simulink model "ControlDes"  (R2026a)
settings: Solver=ode3  StopTime=4  FixedStep=0.001  EnableMultiTasking=on
(part 8 of 12)

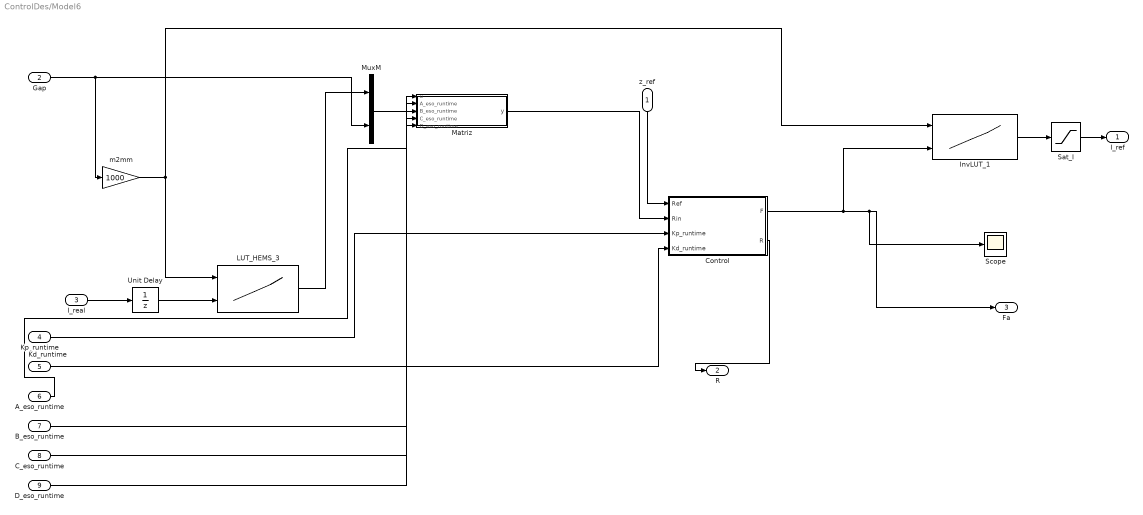
== system ControlDes/Model6 ==
  z_ref : Inport
  Gap : Inport  Port=2
  I_real : Inport  Port=3
  Kp_runtime : Inport  Port=4  OutDataTypeStr=double
  Kd_runtime : Inport  Port=5  OutDataTypeStr=double
  A_eso_runtime : Inport  Port=6  OutDataTypeStr=double  PortDimensions=[3 3]
  B_eso_runtime : Inport  Port=7  OutDataTypeStr=double  PortDimensions=[3 2]
  C_eso_runtime : Inport  Port=8  OutDataTypeStr=double  PortDimensions=[3 3]
  D_eso_runtime : Inport  Port=9  OutDataTypeStr=double  PortDimensions=[3 2]
  Control : Subsystem
  InvLUT_1 : Lookup_n-D  BreakpointsForDimension1=[0.5 1 1.5 2 2.5 3 3.5 4 4.5 5 5.5 6 6.5 7 7.5 8 8.5 9 9.5 10 10.5 11 11.5 12 12.5 13 13.5 14 14.5 15 15.5 16 16.5]  BreakpointsForDimension2=[0 38.719701974874376 77.439403949748751 116.15910592462312 154.8788078994975 193.59850987437187 232.31821184924624 271.03791382412061 309.757615798995 348.47731777386934 387.19701974874374 425.91672172361808 464.63642369849248 503.35612567336682 542.07582764824122 580.79552962311561 619.51523159799001 658.23493357286429 696.95463554773869 735.67433752261297 774.39403949748748 813.11374147236188 851.83344344723616 890.55314542211056 929.27284739698496 967.99254937185924 1006.7122513467336 1045.431953321608 1084.1516552964824 1122.8713572713568 1161.5910592462312 1200.3107612211056 1239.03046319598 1277.7501651708544 1316.4698671457286 1355.189569120603 1393.9092710954774 1432.628973070352 1471.3486750452259 1510.0683770201006 1548.788078994975 1587.5077809698494 1626.2274829447238 1664.9471849195982 1703.6668868944723 1742.3865888693467 1781.1062908442211 1819.8259928190955 1858.5456947939699 1897.2653967688443 1935.9850987437185 1974.7048007185929 2013.4245026934673 2052.1442046683419 2090.8639066432161 2129.5836086180907 2168.3033105929649 2207.023012567839 2245.7427145427137 2284.4624165175878 2323.1821184924625 2361.9018204673371 2400.6215224422112 2439.3412244170854 2478.06092639196 2516.7806283668342 2555.5003303417088 2594.220032316583 2632.9397342914572 2671.6594362663318 2710.379138241206 2749.0988402160806 2787.8185421909548 2826.5382441658294 2865.257946140704 2903.9776481155782 2942.6973500904519 2981.4170520653265 3020.1367540402011 3058.8564560150753 3097.5761579899499 3136.2958599648241 3175.0155619396987 3213.7352639145729 3252.4549658894475 3291.1746678643217 3329.8943698391963 3368.6140718140709 3407.3337737889447 3446.0534757638188 3484.7731777386934 3523.4928797135676 3562.2125816884422 3600.9322836633169 3639.651985638191 3678.3716876130657 3717.0913895879398 3755.8110915628145 3794.5307935376886 3833.2504955125628 3871.970197487437 3910.6898994623116 3949.4096014371858 3988.1293034120604 4026.8490053869346 4065.5687073618092 4104.2884093366838 4143.0081113115584 4181.7278132864321 4220.4475152613068 4259.1672172361814 4297.8869192110551 4336.6066211859297 4375.3263231608043 4414.0460251356781 4452.7657271105527 4491.4854290854273 4530.2051310603019 4568.9248330351757 4607.6445350100503 4646.3642369849249 4685.0839389597995 4723.8036409346741 4762.5233429095479 4801.2430448844225 4839.9627468592962 4878.6824488341708 4917.4021508090455 4956.1218527839201 4994.8415547587938 5033.5612567336684 5072.280958708543 5111.0006606834177 5149.7203626582923 5188.440064633166 5227.1597666080397 5265.8794685829143 5304.5991705577899 5343.3188725326636 5382.0385745075382 5420.7582764824119 5459.4779784572856 5498.1976804321612 5536.9173824070349 5575.6370843819095 5614.3567863567841 5653.0764883316588 5691.7961903065325 5730.515892281408 5769.2355942562817 5807.9552962311564 5846.6749982060301 5885.3947001809038 5924.1144021557793 5962.834104130653 6001.5538061055277 6040.2735080804023 6078.9932100552769 6117.7129120301506 6156.4326140050252 6195.1523159798999 6233.8720179547745 6272.5917199296482 6311.3114219045219 6350.0311238793975 6388.7508258542712 6427.4705278291458 6466.1902298040195 6504.909931778895 6543.6296337537688 6582.3493357286434 6621.069037703518 6659.7887396783926 6698.5084416532663 6737.2281436281419 6775.9478456030156 6814.6675475778893 6853.3872495527639 6892.1069515276376 6930.8266535025132 6969.5463554773869 7008.2660574522615 7046.9857594271352 7085.7054614020108 7124.4251633768845 7163.1448653517591 7201.8645673266337 7240.5842693015074 7279.3039712763821 7318.0236732512558 7356.7433752261313 7395.463077201005 7434.1827791758797 7472.9024811507534 7511.6221831256289 7550.3418851005026 7589.0615870753772 7627.7812890502519 7666.5009910251256 7705.2206930000002]  Table=[0 0.20825445101853096 0.41650890203706192 0.62476335305559283 0.83301780407412385 1.0135826468062146 1.082118922511446 1.1506551982166775 1.219191473921909 1.2877277496271402 1.3562640253323717 1.4248003010376031 1.4933365767428346 1.5618728524480658 1.6304091281532973 1.6989454038585288 1.7674816795637602 1.8360179552689915 1.9045542309742229 1.9730905066794542 2.0259914205399863 2.0687849073782689 2.1115783942165511 2.1543718810548338 2.1971653678931164 2.2399588547313991 2.2827523415696813 2.325545828407964 2.3683393152462466 2.4111328020845288 2.4539262889228119 2.4967197757610946 2.5395132625993773 2.5823067494376595 2.6251002362759417 2.6678937231142243 2.710687209952507 2.7534806967907901 2.7962741836290719 2.839067670467355 2.8818611573056376 2.9246546441439203 2.9674481309822025 3.0082039458877476 3.0424832420422163 3.076762538196685 3.1110418343511541 3.1453211305056232 3.1796004266600919 3.2138797228145606 3.2481590189690297 3.2824383151234988 3.3167176112779675 3.3509969074324366 3.3852762035869057 3.4195554997413744 3.4538347958958431 3.4881140920503118 3.5223933882047813 3.55667268435925 3.5909519805137191 3.6252312766681882 3.6595105728226569 3.6937898689771256 3.7280691651315947 3.7623484612860634 3.7966277574405325 3.8309070535950012 3.8651863497494698 3.8994656459039394 3.9337449420584081 3.9680242382128772 4.0026883536532365 4.0426942126296082 4.0827000716059798 4.1227059305823506 4.1627117895587222 4.2027176485350939 4.2427235075114647 4.2827293664878363 4.3227352254642071 4.3627410844405787 4.4027469434169504 4.4427528023933212 4.4827586613696928 4.5227645203460636 4.5627703793224352 4.6027762382988069 4.6427820972751777 4.6827879562515484 4.7227938152279201 4.7627996742042917 4.8028055331806625 4.842811392157035 4.8828172511334049 4.9228231101097766 4.9628289690861482 5.004895171693434 5.0739771562489926 5.1430591408045503 5.212141125360108 5.2812231099156675 5.350305094471226 5.4193870790267855 5.4884690635823423 5.5575510481379027 5.6266330326934613 5.6957150172490207 5.7647970018045775 5.8338789863601361 5.9029609709156956 5.9720429554712533 6.060635964208382 6.1624927143999662 6.2643494645915485 6.3662062147831326 6.4680629649747168 6.5699197151663018 6.6717764653578833 6.7736332155494674 6.8754899657410515 6.9773467159326366 7.1052458067439899 7.2405933662740365 7.3759409258040867 7.5112884853341342 7.6466360448641844 7.7819836043942345 7.9173311639242847 8.0581390909222392 8.2075159845450063 8.3568928781677734 8.5062697717905404 8.6556466654133075 8.8050235590360693 8.9544004526588328 9.1109942620640414 9.2707591690610673 9.430524076058088 9.5902889830551104 9.7500538900521292 9.909818797049148 10.07860600232517 10.259086199851795 10.439566397378425 10.620046594905055 10.800526792431686 10.981006989958312 11.179637509673544 11.380402745194747 11.581167980715957 11.781933216237162 11.982698451758367 12.200814130096445 12.420566042437333 12.640317954778226 12.860069867119119 13.126007972843706 13.472911953059718 13.819815933275743 14.248324772175067 14.765028806201716 15.318870467347217 15.903685701086824 16.530613286533896 17.178435440269205 17.861895428989815 18.58639634639496 19.342319000305999 20.130582236557807 20.946504242050416 21.793465366913725 22.66596895426494 23.559530190599418 24.471656612462336 25.40419986962144 26.362632409957975 27.351818955653389 28.373533575187398 29.440672985292188 30.570327923183555 31.757263294366073 32.986746804015425 34.246450693164164 35.52223706959721 36.807114490416751 38.099172703380667 39.396598812923777 40.695909456634084 41.995762806636158 43.296542367305818 44.597395639785859 45.898496497631839 47.199521876773268 48.499918470691156 49.80095993571296 51.101605949724835 52.401915628484389 53.701245517447497 55;0 0.76888357898292115 1.1751199837457729 1.4255013576533873 1.6758827315610019 1.9262641054686163 2.1058823348051132 2.2559623966027069 2.4060424584003006 2.5561225201978948 2.706202581995488 2.8562826437930822 3.0045785783675409 3.1125756111632508 ...(+52833 chars)]  ExtrapMethod=Clip  InternalRulePriority=Speed  RndMeth=Simplest
      settings: InputPortMap=u0,u1
  LUT_HEMS_3 : Lookup_n-D  BreakpointsForDimension1=[0.5 1 1.5 2 2.5 3 3.5 4 4.5 5 5.5 6 6.5 7 7.5 8 8.5 9 9.5 10 10.5 11 11.5 12 12.5 13 13.5 14 14.5 15 15.5 16 16.5]  BreakpointsForDimension2=[0 1 2 3 4 5 6 7 8 9 10 11 12 13 14 15 16 17 18 19 20 21 22 23 24 25 26 27 28 29 30 31 32 33 34 35 36 37 38 39 40 41 42 43 44 45 46 47 48 49 50 51 52 53 54 55]  Table=[0 185.9249672 750.87690799999996 1655.6805320000001 2785.216617 3753.0674009999998 4313.5565390000002 4693.6953309999999 4979.7714310000001 5238.9795389999999 5481.3337750000001 5695.8708960000004 5888.731487 6064.928825 6176.543866 6251.4798049999999 6317.6882409999998 6378.6420159999998 6435.2944939999998 6487.981957 6537.4328340000002 6584.8879850000003 6630.4867649999997 6674.4857750000001 6717.4194129999996 6759.4176170000001 6800.3137919999999 6839.8959009999999 6878.2433190000002 6915.358142 6950.460161 6983.9254600000004 7016.0683060000001 7047.4010179999996 7078.2087309999997 7108.6275150000001 7138.8774709999998 7168.9443259999998 7198.9040859999996 7228.755862 7258.5804779999999 7288.3594860000003 7318.1499009999998 7347.9142069999998 7377.6879230000004 7407.4423319999996 7437.2036580000004 7466.9636659999996 7496.7288989999997 7526.5203250000004 7556.2615880000003 7586.0370910000001 7615.8040099999998 7645.6044910000001 7675.4036120000001 7705.2206930000002;0 50.358341670000001 205.00124249999999 462.99488609999997 821.52049529999999 1275.4488719999999 1815.4468879999999 2417.3712139999998 3013.984723 3491.2876780000001 3838.5691499999998 4118.0858349999999 4346.8618219999998 4558.9346269999996 4759.0309299999999 4942.0177089999997 5105.9639639999996 5253.0348219999996 5362.5162200000004 5440.8379949999999 5509.7998870000001 5572.7200860000003 5632.2593720000004 5689.6635800000004 5744.5173999999997 5797.501671 5848.7229440000001 5898.1835080000001 5945.531156 5990.6949679999998 6033.8417140000001 6075.4827839999998 6116.2033110000002 6156.1693610000002 6195.5075500000003 6234.0945689999999 6271.969083 6309.1572560000004 6345.8601040000003 6382.0602360000003 6417.9799970000004 6453.7335750000002 6489.4389899999996 6524.967318 6560.4583140000004 6595.8979929999996 6631.2596970000004 6666.589696 6701.9197940000004 6737.2543530000003 6772.5132160000003 6807.4936710000002 6842.7713949999998 6878.0320149999998 6913.2557580000002 6948.244514;0 23.217442720000001 94.340941790000002 213.54810789999999 380.32169820000001 594.10779100000002 853.75137949999998 1157.775693 1503.429785 1885.7072029999999 2292.655694 2695.2178359999998 3047.2340450000002 3333.626076 3570.0121479999998 3775.3560849999999 3956.766744 4130.4705430000004 4294.9133119999997 4445.6965689999997 4581.0417340000004 4698.4210039999998 4781.1550289999996 4850.4790350000003 4914.313545 4973.7074190000003 5029.9002440000004 5083.9691949999997 5136.4099939999996 5187.3495039999998 5236.6530620000003 5284.2207799999996 5330.4212090000001 5374.8830310000003 5418.0854280000003 5460.1024360000001 5500.9334369999997 5540.6684009999999 5579.5738739999997 5617.6247839999996 5655.3618999999999 5692.4378129999996 5729.1741149999998 5765.5516250000001 5801.609152 5837.3326639999996 5872.7456380000003 5907.7882120000004 5942.4348559999999 5976.8747679999997 6011.116575 6045.2074650000004 6079.1768570000004 6113.0063190000001 6146.7426459999997 6180.3508119999997;0 13.53731471 54.920810189999997 124.2975659 221.6197512 346.61976329999999 499.12409639999998 678.70434439999997 884.82418110000003 1116.8384940000001 1373.3669870000001 1652.3955370000001 1949.420372 2255.209852 2551.5274100000001 2814.929267 3040.2881179999999 3235.3113589999998 3409.6099049999998 3565.7882319999999 3715.897301 3859.331279 3993.5367590000001 4113.8205090000001 4220.3495819999998 4301.0390870000001 4365.2183219999997 4425.1897019999997 4481.4847470000004 4535.2844709999999 4586.646702 4636.465835 4684.7545060000002 4731.7352920000003 4777.4680070000004 4822.0362409999998 4864.7284479999998 4905.8761789999999 4946.3990480000002 4985.9961940000003 5025.0588399999997 5063.5062950000001 5101.2281560000001 5137.8316869999999 5174.0463900000004 5209.788939 5245.1148999999996 5279.904544 5314.3628760000001 5348.6515650000001 5382.7712929999998 5416.7071859999996 5450.5303219999996 5484.1124309999996 5517.5429899999999 5550.8569729999999;0 9.0480587680000006 36.63580752 82.898906339999996 ...(+27351 chars)]  ExtrapMethod=Clip  InternalRulePriority=Speed  RndMeth=Simplest
      settings: InputPortMap=u0,u1
  Matriz : Subsystem
  MuxM : Mux  Inputs=2
  Sat_I : Saturate  UpperLimit=50  LowerLimit=-50
  Scope : Scope
      settings: ActiveDisplayYMinimum=-11967.729581091611  ActiveDisplayYMaximum=16975.635504075348  DataLoggingVariableName=ScopeData6
  Unit Delay : UnitDelay  SampleTime=-1
  m2mm : Gain  Gain=1000
  I_ref : Outport
  R : Outport  Port=2
  Fa : Outport  Port=3
  wires:
  LUT_HEMS_3/1 -> MuxM/1
  Sat_I/1 -> I_ref/1
  InvLUT_1/1 -> Sat_I/1
  Unit Delay/1 -> LUT_HEMS_3/2
  m2mm/1 -> InvLUT_1/1, LUT_HEMS_3/1
  Gap/1 -> m2mm/1, MuxM/2
  I_real/1 -> Unit Delay/1
  MuxM/1 -> Matriz/1(u)
  z_ref/1 -> Control/1(Ref)
  Matriz/1(y) -> Control/2(Rin)
  Control/1(F) -> InvLUT_1/2, Scope/1, Fa/1
  Control/2(R) -> R/1
  Kp_runtime/1 -> Control/3(Kp_runtime)
  Kd_runtime/1 -> Control/4(Kd_runtime)
  A_eso_runtime/1 -> Matriz/2(A_eso_runtime)
  B_eso_runtime/1 -> Matriz/3(B_eso_runtime)
  C_eso_runtime/1 -> Matriz/4(C_eso_runtime)
  D_eso_runtime/1 -> Matriz/5(D_eso_runtime)
